simulink model "Mux8Bit4To1"  (R2014a)
settings: Solver=ode45  StartTime=0.0  StopTime=10.0  RelTol=1e-3
libraries: hdlsllib x35
settings Model: Creator=you.r  LastModifiedBy=you.r

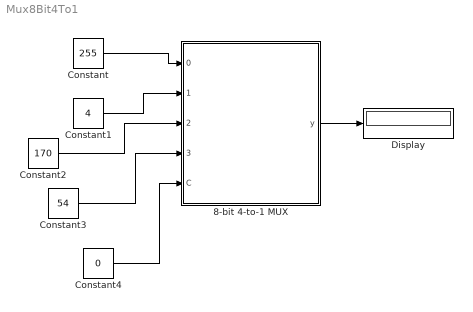
== system Mux8Bit4To1 ==
  8-bit 4-to-1 MUX : Subsystem
  Constant : Constant  Value=255  OutDataTypeStr=uint8  SampleTime=1
  Constant1 : Constant  Value=4  OutDataTypeStr=uint8  SampleTime=1
  Constant2 : Constant  Value=170  OutDataTypeStr=uint8  SampleTime=1
  Constant3 : Constant  Value=54  OutDataTypeStr=uint8  SampleTime=1
  Constant4 : Constant  Value=0  OutDataTypeStr=uint8  SampleTime=1
  Display : Display
  wires:
  Constant/1 -> 8-bit 4-to-1 MUX/1(0)
  Constant1/1 -> 8-bit 4-to-1 MUX/2(1)
  Constant2/1 -> 8-bit 4-to-1 MUX/3(2)
  Constant3/1 -> 8-bit 4-to-1 MUX/4(3)
  Constant4/1 -> 8-bit 4-to-1 MUX/5(C)
  8-bit 4-to-1 MUX/1(y) -> Display/1

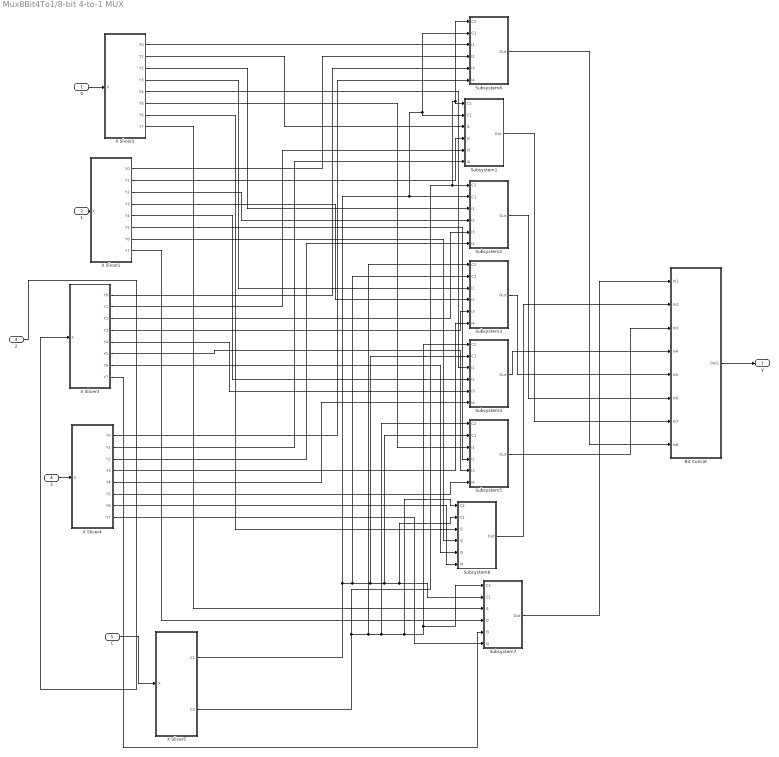
== system Mux8Bit4To1/8-bit 4-to-1 MUX ==
  0 : Inport  OutDataTypeStr=uint8  SampleTime=1
  1 : Inport  Port=2  OutDataTypeStr=uint8  SampleTime=1
  2 : Inport  Port=3  OutDataTypeStr=uint8  SampleTime=1
  3 : Inport  Port=4  OutDataTypeStr=uint8  SampleTime=1
  C : Inport  Port=5  OutDataTypeStr=uint8  SampleTime=1
  Bit Concat : Subsystem
  Subsystem1 : Subsystem
  Subsystem2 : Subsystem
  Subsystem3 : Subsystem
  Subsystem4 : Subsystem
  Subsystem5 : Subsystem
  Subsystem6 : Subsystem
  Subsystem7 : Subsystem
  Subsystem8 : Subsystem
  X Slicer1 : Subsystem
  X Slicer2 : Subsystem
  X Slicer3 : Subsystem
  X Slicer4 : Subsystem
  X Slicer5 : Subsystem
  y : Outport  SampleTime=1
  wires:
  X Slicer1/4(Y3) -> Subsystem3/4(I2)
  1/1 -> X Slicer1/1(X)
  X Slicer3/2(Y1) -> Subsystem1/5(I3)
  X Slicer4/4(Y3) -> Subsystem3/6(I4)
  X Slicer1/1(Y0) -> Subsystem8/4(I2)
  X Slicer1/2(Y1) -> Subsystem1/4(I2)
  X Slicer2/3(Y2) -> Subsystem2/3(I1)
  X Slicer5/2(C2) -> Subsystem2/1(C2), Subsystem1/1(C2), Subsystem8/1(C2), Subsystem3/1(C2), Subsystem5/1(C2), Subsystem6/1(C2), Subsystem7/1(C2), Subsystem4/1(C2)
  X Slicer1/3(Y2) -> Subsystem2/4(I2)
  X Slicer3/7(Y6) -> Subsystem6/5(I3)
  X Slicer2/2(Y1) -> Subsystem1/3(I1)
  X Slicer5/1(C1) -> Subsystem2/2(C1), Subsystem1/2(C1), Subsystem8/2(C1), Subsystem3/2(C1), Subsystem4/2(C1), Subsystem5/2(C1), Subsystem7/2(C1), Subsystem6/2(C1)
  X Slicer4/1(Y0) -> Subsystem8/6(I4)
  0/1 -> X Slicer2/1(X)
  X Slicer3/1(Y0) -> Subsystem8/5(I3)
  X Slicer1/8(Y7) -> Subsystem7/4(I2)
  X Slicer1/5(Y4) -> Subsystem4/4(I2)
  X Slicer3/6(Y5) -> Subsystem5/5(I3)
  X Slicer4/2(Y1) -> Subsystem1/6(I4)
  X Slicer2/6(Y5) -> Subsystem5/3(I1)
  X Slicer4/6(Y5) -> Subsystem5/6(I4)
  X Slicer1/6(Y5) -> Subsystem5/4(I2)
  X Slicer2/1(Y0) -> Subsystem8/3(I1)
  X Slicer4/3(Y2) -> Subsystem2/6(I4)
  X Slicer2/5(Y4) -> Subsystem4/3(I1)
  2/1 -> X Slicer3/1(X)
  3/1 -> X Slicer4/1(X)
  X Slicer1/7(Y6) -> Subsystem6/4(I2)
  Bit Concat/1(Out1) -> y/1
  X Slicer4/7(Y6) -> Subsystem6/6(I4)
  X Slicer3/5(Y4) -> Subsystem4/5(I3)
  X Slicer2/7(Y6) -> Subsystem6/3(I1)
  C/1 -> X Slicer5/1(X)
  X Slicer2/4(Y3) -> Subsystem3/3(I1)
  X Slicer4/5(Y4) -> Subsystem4/6(I4)
  X Slicer3/4(Y3) -> Subsystem3/5(I3)
  X Slicer4/8(Y7) -> Subsystem7/6(I4)
  X Slicer3/8(Y7) -> Subsystem7/5(I3)
  Subsystem2/1(Out) -> Bit Concat/6(In6)
  Subsystem1/1(Out) -> Bit Concat/7(In7)
  Subsystem8/1(Out) -> Bit Concat/8(In8)
  Subsystem3/1(Out) -> Bit Concat/5(In5)
  Subsystem6/1(Out) -> Bit Concat/2(In2)
  Subsystem4/1(Out) -> Bit Concat/4(In4)
  Subsystem5/1(Out) -> Bit Concat/3(In3)
  Subsystem7/1(Out) -> Bit Concat/1(In1)
  X Slicer2/8(Y7) -> Subsystem7/3(I1)
  X Slicer3/3(Y2) -> Subsystem2/5(I3)

== system Mux8Bit4To1/8-bit 4-to-1 MUX/Bit Concat ==
  In1 : Inport
  In2 : Inport  Port=2
  In3 : Inport  Port=3
  In4 : Inport  Port=4
  In5 : Inport  Port=5
  In6 : Inport  Port=6
  In7 : Inport  Port=7
  In8 : Inport  Port=8
  Bit Concat : hdlsllib/HDL Operations/Bit Concat  numInputs=8
  Data Type Conversion : DataTypeConversion  OutDataTypeStr=uint16
  Out1 : Outport
  wires:
  Data Type Conversion/1 -> Out1/1
  Bit Concat/1 -> Data Type Conversion/1
  In7/1 -> Bit Concat/7
  In1/1 -> Bit Concat/1
  In8/1 -> Bit Concat/8
  In6/1 -> Bit Concat/6
  In2/1 -> Bit Concat/2
  In5/1 -> Bit Concat/5
  In3/1 -> Bit Concat/3
  In4/1 -> Bit Concat/4

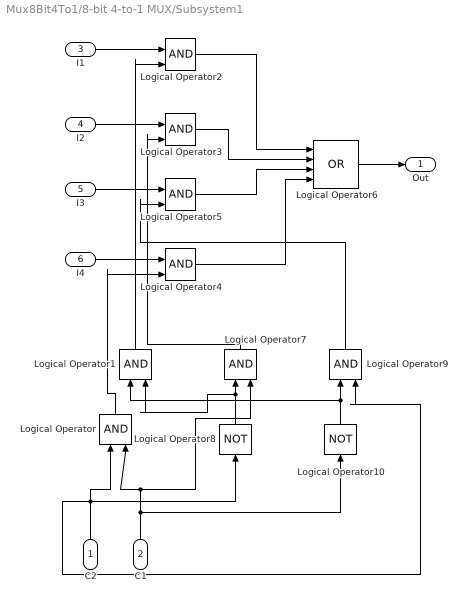
== system Mux8Bit4To1/8-bit 4-to-1 MUX/Subsystem1 ==
  C2 : Inport
  C1 : Inport  Port=2
  I1 : Inport  Port=3
  I2 : Inport  Port=4
  I3 : Inport  Port=5
  I4 : Inport  Port=6
  Logical Operator{,1..5,7,9} (8 alike) : Logic  IconShape=distinctive  AllPortsSameDT=off  OutDataTypeStr=boolean
  Logical Operator10 : Logic  Operator=NOT  IconShape=distinctive  AllPortsSameDT=off  OutDataTypeStr=boolean
  Logical Operator6 : Logic  Operator=OR  Inputs=4  IconShape=distinctive  AllPortsSameDT=off  OutDataTypeStr=boolean
  Logical Operator8 : Logic  Operator=NOT  IconShape=distinctive  AllPortsSameDT=off  OutDataTypeStr=boolean
  Out : Outport
  wires:
  I1/1 -> Logical Operator2/1
  I3/1 -> Logical Operator5/1
  Logical Operator4/1 -> Logical Operator6/4
  Logical Operator3/1 -> Logical Operator6/2
  C1/1 -> Logical Operator10/1, Logical Operator/2, Logical Operator7/2
  C2/1 -> Logical Operator9/2, Logical Operator/1, Logical Operator8/1
  Logical Operator10/1 -> Logical Operator1/1, Logical Operator9/1
  Logical Operator/1 -> Logical Operator4/2
  Logical Operator7/1 -> Logical Operator3/2
  I2/1 -> Logical Operator3/1
  Logical Operator2/1 -> Logical Operator6/1
  Logical Operator9/1 -> Logical Operator5/2
  I4/1 -> Logical Operator4/1
  Logical Operator5/1 -> Logical Operator6/3
  Logical Operator6/1 -> Out/1
  Logical Operator8/1 -> Logical Operator1/2, Logical Operator7/1
  Logical Operator1/1 -> Logical Operator2/2

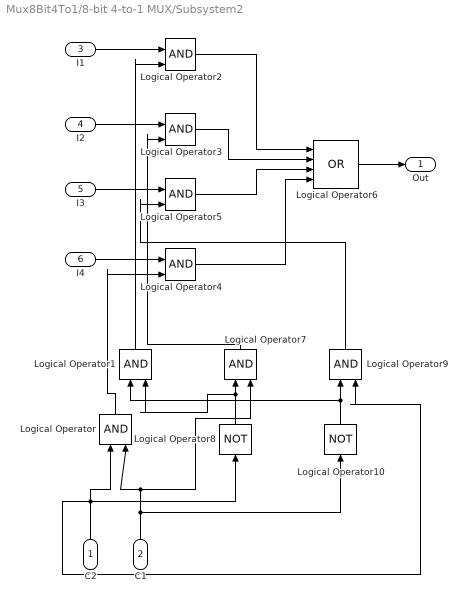
== system Mux8Bit4To1/8-bit 4-to-1 MUX/Subsystem2 ==
  C2 : Inport
  C1 : Inport  Port=2
  I1 : Inport  Port=3
  I2 : Inport  Port=4
  I3 : Inport  Port=5
  I4 : Inport  Port=6
  Logical Operator{,1..5,7,9} (8 alike) : Logic  IconShape=distinctive  AllPortsSameDT=off  OutDataTypeStr=boolean
  Logical Operator10 : Logic  Operator=NOT  IconShape=distinctive  AllPortsSameDT=off  OutDataTypeStr=boolean
  Logical Operator6 : Logic  Operator=OR  Inputs=4  IconShape=distinctive  AllPortsSameDT=off  OutDataTypeStr=boolean
  Logical Operator8 : Logic  Operator=NOT  IconShape=distinctive  AllPortsSameDT=off  OutDataTypeStr=boolean
  Out : Outport
  wires:
  I1/1 -> Logical Operator2/1
  I3/1 -> Logical Operator5/1
  Logical Operator4/1 -> Logical Operator6/4
  Logical Operator3/1 -> Logical Operator6/2
  C1/1 -> Logical Operator10/1, Logical Operator/2, Logical Operator7/2
  C2/1 -> Logical Operator9/2, Logical Operator/1, Logical Operator8/1
  Logical Operator10/1 -> Logical Operator1/1, Logical Operator9/1
  Logical Operator/1 -> Logical Operator4/2
  Logical Operator7/1 -> Logical Operator3/2
  I2/1 -> Logical Operator3/1
  Logical Operator2/1 -> Logical Operator6/1
  Logical Operator9/1 -> Logical Operator5/2
  I4/1 -> Logical Operator4/1
  Logical Operator5/1 -> Logical Operator6/3
  Logical Operator6/1 -> Out/1
  Logical Operator8/1 -> Logical Operator1/2, Logical Operator7/1
  Logical Operator1/1 -> Logical Operator2/2

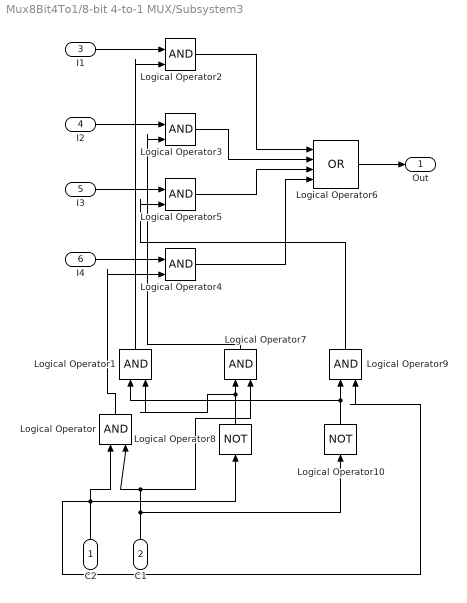
== system Mux8Bit4To1/8-bit 4-to-1 MUX/Subsystem3 ==
  C2 : Inport
  C1 : Inport  Port=2
  I1 : Inport  Port=3
  I2 : Inport  Port=4
  I3 : Inport  Port=5
  I4 : Inport  Port=6
  Logical Operator{,1..5,7,9} (8 alike) : Logic  IconShape=distinctive  AllPortsSameDT=off  OutDataTypeStr=boolean
  Logical Operator10 : Logic  Operator=NOT  IconShape=distinctive  AllPortsSameDT=off  OutDataTypeStr=boolean
  Logical Operator6 : Logic  Operator=OR  Inputs=4  IconShape=distinctive  AllPortsSameDT=off  OutDataTypeStr=boolean
  Logical Operator8 : Logic  Operator=NOT  IconShape=distinctive  AllPortsSameDT=off  OutDataTypeStr=boolean
  Out : Outport
  wires:
  I1/1 -> Logical Operator2/1
  I3/1 -> Logical Operator5/1
  Logical Operator4/1 -> Logical Operator6/4
  Logical Operator3/1 -> Logical Operator6/2
  C1/1 -> Logical Operator10/1, Logical Operator/2, Logical Operator7/2
  C2/1 -> Logical Operator9/2, Logical Operator/1, Logical Operator8/1
  Logical Operator10/1 -> Logical Operator1/1, Logical Operator9/1
  Logical Operator/1 -> Logical Operator4/2
  Logical Operator7/1 -> Logical Operator3/2
  I2/1 -> Logical Operator3/1
  Logical Operator2/1 -> Logical Operator6/1
  Logical Operator9/1 -> Logical Operator5/2
  I4/1 -> Logical Operator4/1
  Logical Operator5/1 -> Logical Operator6/3
  Logical Operator6/1 -> Out/1
  Logical Operator8/1 -> Logical Operator1/2, Logical Operator7/1
  Logical Operator1/1 -> Logical Operator2/2

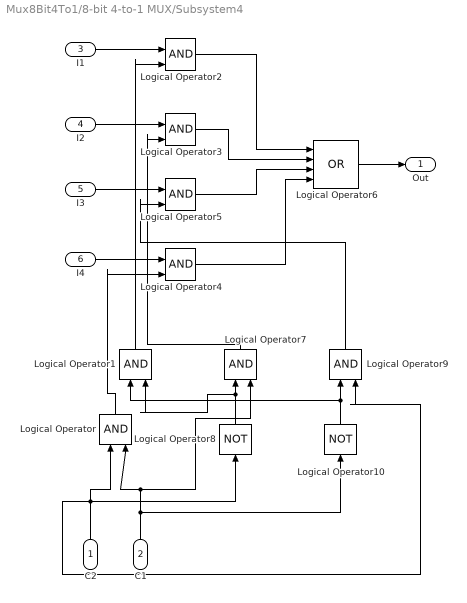
== system Mux8Bit4To1/8-bit 4-to-1 MUX/Subsystem4 ==
  C2 : Inport
  C1 : Inport  Port=2
  I1 : Inport  Port=3
  I2 : Inport  Port=4
  I3 : Inport  Port=5
  I4 : Inport  Port=6
  Logical Operator{,1..5,7,9} (8 alike) : Logic  IconShape=distinctive  AllPortsSameDT=off  OutDataTypeStr=boolean
  Logical Operator10 : Logic  Operator=NOT  IconShape=distinctive  AllPortsSameDT=off  OutDataTypeStr=boolean
  Logical Operator6 : Logic  Operator=OR  Inputs=4  IconShape=distinctive  AllPortsSameDT=off  OutDataTypeStr=boolean
  Logical Operator8 : Logic  Operator=NOT  IconShape=distinctive  AllPortsSameDT=off  OutDataTypeStr=boolean
  Out : Outport
  wires:
  I1/1 -> Logical Operator2/1
  I3/1 -> Logical Operator5/1
  Logical Operator4/1 -> Logical Operator6/4
  Logical Operator3/1 -> Logical Operator6/2
  C1/1 -> Logical Operator10/1, Logical Operator/2, Logical Operator7/2
  C2/1 -> Logical Operator9/2, Logical Operator/1, Logical Operator8/1
  Logical Operator10/1 -> Logical Operator1/1, Logical Operator9/1
  Logical Operator/1 -> Logical Operator4/2
  Logical Operator7/1 -> Logical Operator3/2
  I2/1 -> Logical Operator3/1
  Logical Operator2/1 -> Logical Operator6/1
  Logical Operator9/1 -> Logical Operator5/2
  I4/1 -> Logical Operator4/1
  Logical Operator5/1 -> Logical Operator6/3
  Logical Operator6/1 -> Out/1
  Logical Operator8/1 -> Logical Operator1/2, Logical Operator7/1
  Logical Operator1/1 -> Logical Operator2/2

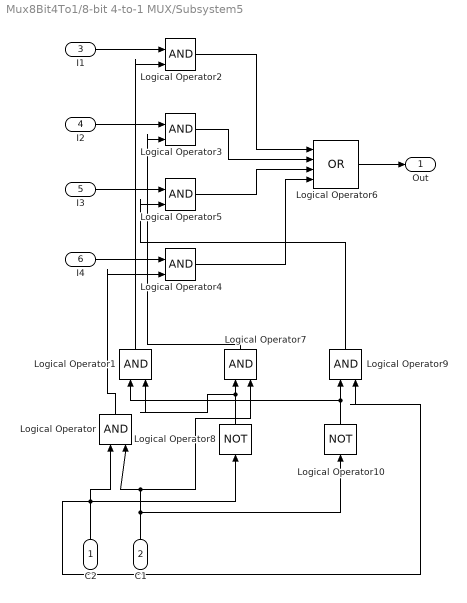
== system Mux8Bit4To1/8-bit 4-to-1 MUX/Subsystem5 ==
  C2 : Inport
  C1 : Inport  Port=2
  I1 : Inport  Port=3
  I2 : Inport  Port=4
  I3 : Inport  Port=5
  I4 : Inport  Port=6
  Logical Operator{,1..5,7,9} (8 alike) : Logic  IconShape=distinctive  AllPortsSameDT=off  OutDataTypeStr=boolean
  Logical Operator10 : Logic  Operator=NOT  IconShape=distinctive  AllPortsSameDT=off  OutDataTypeStr=boolean
  Logical Operator6 : Logic  Operator=OR  Inputs=4  IconShape=distinctive  AllPortsSameDT=off  OutDataTypeStr=boolean
  Logical Operator8 : Logic  Operator=NOT  IconShape=distinctive  AllPortsSameDT=off  OutDataTypeStr=boolean
  Out : Outport
  wires:
  I1/1 -> Logical Operator2/1
  I3/1 -> Logical Operator5/1
  Logical Operator4/1 -> Logical Operator6/4
  Logical Operator3/1 -> Logical Operator6/2
  C1/1 -> Logical Operator10/1, Logical Operator/2, Logical Operator7/2
  C2/1 -> Logical Operator9/2, Logical Operator/1, Logical Operator8/1
  Logical Operator10/1 -> Logical Operator1/1, Logical Operator9/1
  Logical Operator/1 -> Logical Operator4/2
  Logical Operator7/1 -> Logical Operator3/2
  I2/1 -> Logical Operator3/1
  Logical Operator2/1 -> Logical Operator6/1
  Logical Operator9/1 -> Logical Operator5/2
  I4/1 -> Logical Operator4/1
  Logical Operator5/1 -> Logical Operator6/3
  Logical Operator6/1 -> Out/1
  Logical Operator8/1 -> Logical Operator1/2, Logical Operator7/1
  Logical Operator1/1 -> Logical Operator2/2

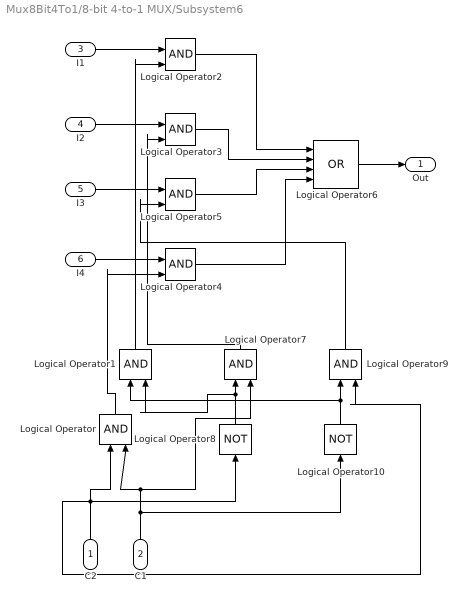
== system Mux8Bit4To1/8-bit 4-to-1 MUX/Subsystem6 ==
  C2 : Inport
  C1 : Inport  Port=2
  I1 : Inport  Port=3
  I2 : Inport  Port=4
  I3 : Inport  Port=5
  I4 : Inport  Port=6
  Logical Operator{,1..5,7,9} (8 alike) : Logic  IconShape=distinctive  AllPortsSameDT=off  OutDataTypeStr=boolean
  Logical Operator10 : Logic  Operator=NOT  IconShape=distinctive  AllPortsSameDT=off  OutDataTypeStr=boolean
  Logical Operator6 : Logic  Operator=OR  Inputs=4  IconShape=distinctive  AllPortsSameDT=off  OutDataTypeStr=boolean
  Logical Operator8 : Logic  Operator=NOT  IconShape=distinctive  AllPortsSameDT=off  OutDataTypeStr=boolean
  Out : Outport
  wires:
  I1/1 -> Logical Operator2/1
  I3/1 -> Logical Operator5/1
  Logical Operator4/1 -> Logical Operator6/4
  Logical Operator3/1 -> Logical Operator6/2
  C1/1 -> Logical Operator10/1, Logical Operator/2, Logical Operator7/2
  C2/1 -> Logical Operator9/2, Logical Operator/1, Logical Operator8/1
  Logical Operator10/1 -> Logical Operator1/1, Logical Operator9/1
  Logical Operator/1 -> Logical Operator4/2
  Logical Operator7/1 -> Logical Operator3/2
  I2/1 -> Logical Operator3/1
  Logical Operator2/1 -> Logical Operator6/1
  Logical Operator9/1 -> Logical Operator5/2
  I4/1 -> Logical Operator4/1
  Logical Operator5/1 -> Logical Operator6/3
  Logical Operator6/1 -> Out/1
  Logical Operator8/1 -> Logical Operator1/2, Logical Operator7/1
  Logical Operator1/1 -> Logical Operator2/2

== system Mux8Bit4To1/8-bit 4-to-1 MUX/Subsystem7 ==
  C2 : Inport
  C1 : Inport  Port=2
  I1 : Inport  Port=3
  I2 : Inport  Port=4
  I3 : Inport  Port=5
  I4 : Inport  Port=6
  Logical Operator{,1..5,7,9} (8 alike) : Logic  IconShape=distinctive  AllPortsSameDT=off  OutDataTypeStr=boolean
  Logical Operator10 : Logic  Operator=NOT  IconShape=distinctive  AllPortsSameDT=off  OutDataTypeStr=boolean
  Logical Operator6 : Logic  Operator=OR  Inputs=4  IconShape=distinctive  AllPortsSameDT=off  OutDataTypeStr=boolean
  Logical Operator8 : Logic  Operator=NOT  IconShape=distinctive  AllPortsSameDT=off  OutDataTypeStr=boolean
  Out : Outport
  wires:
  I1/1 -> Logical Operator2/1
  I3/1 -> Logical Operator5/1
  Logical Operator4/1 -> Logical Operator6/4
  Logical Operator3/1 -> Logical Operator6/2
  C1/1 -> Logical Operator10/1, Logical Operator/2, Logical Operator7/2
  C2/1 -> Logical Operator9/2, Logical Operator/1, Logical Operator8/1
  Logical Operator10/1 -> Logical Operator1/1, Logical Operator9/1
  Logical Operator/1 -> Logical Operator4/2
  Logical Operator7/1 -> Logical Operator3/2
  I2/1 -> Logical Operator3/1
  Logical Operator2/1 -> Logical Operator6/1
  Logical Operator9/1 -> Logical Operator5/2
  I4/1 -> Logical Operator4/1
  Logical Operator5/1 -> Logical Operator6/3
  Logical Operator6/1 -> Out/1
  Logical Operator8/1 -> Logical Operator1/2, Logical Operator7/1
  Logical Operator1/1 -> Logical Operator2/2

== system Mux8Bit4To1/8-bit 4-to-1 MUX/Subsystem8 ==
  C2 : Inport
  C1 : Inport  Port=2
  I1 : Inport  Port=3
  I2 : Inport  Port=4
  I3 : Inport  Port=5
  I4 : Inport  Port=6
  Logical Operator{,1..5,7,9} (8 alike) : Logic  IconShape=distinctive  AllPortsSameDT=off  OutDataTypeStr=boolean
  Logical Operator10 : Logic  Operator=NOT  IconShape=distinctive  AllPortsSameDT=off  OutDataTypeStr=boolean
  Logical Operator6 : Logic  Operator=OR  Inputs=4  IconShape=distinctive  AllPortsSameDT=off  OutDataTypeStr=boolean
  Logical Operator8 : Logic  Operator=NOT  IconShape=distinctive  AllPortsSameDT=off  OutDataTypeStr=boolean
  Out : Outport
  wires:
  I1/1 -> Logical Operator2/1
  I3/1 -> Logical Operator5/1
  Logical Operator4/1 -> Logical Operator6/4
  Logical Operator3/1 -> Logical Operator6/2
  C1/1 -> Logical Operator10/1, Logical Operator/2, Logical Operator7/2
  C2/1 -> Logical Operator9/2, Logical Operator/1, Logical Operator8/1
  Logical Operator10/1 -> Logical Operator1/1, Logical Operator9/1
  Logical Operator/1 -> Logical Operator4/2
  Logical Operator7/1 -> Logical Operator3/2
  I2/1 -> Logical Operator3/1
  Logical Operator2/1 -> Logical Operator6/1
  Logical Operator9/1 -> Logical Operator5/2
  I4/1 -> Logical Operator4/1
  Logical Operator5/1 -> Logical Operator6/3
  Logical Operator6/1 -> Out/1
  Logical Operator8/1 -> Logical Operator1/2, Logical Operator7/1
  Logical Operator1/1 -> Logical Operator2/2

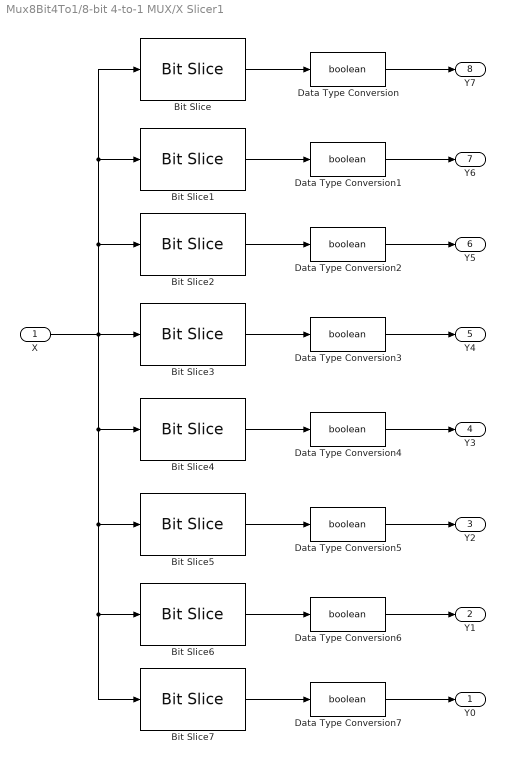
== system Mux8Bit4To1/8-bit 4-to-1 MUX/X Slicer1 ==
  X : Inport  OutDataTypeStr=uint8  SampleTime=1
  Bit Slice : hdlsllib/HDL Operations/Bit Slice  lidx=7  ridx=7
  Bit Slice1 : hdlsllib/HDL Operations/Bit Slice  lidx=6  ridx=6
  Bit Slice2 : hdlsllib/HDL Operations/Bit Slice  lidx=5  ridx=5
  Bit Slice3 : hdlsllib/HDL Operations/Bit Slice  lidx=4  ridx=4
  Bit Slice4 : hdlsllib/HDL Operations/Bit Slice  lidx=3  ridx=3
  Bit Slice5 : hdlsllib/HDL Operations/Bit Slice  lidx=2  ridx=2
  Bit Slice6 : hdlsllib/HDL Operations/Bit Slice  lidx=1  ridx=1
  Bit Slice7 : hdlsllib/HDL Operations/Bit Slice  lidx=0  ridx=0
  Data Type Conversion{,1..7} (8 alike) : DataTypeConversion  OutDataTypeStr=boolean
  Y0 : Outport  OutDataTypeStr=boolean  SampleTime=1
  Y1 : Outport  Port=2  OutDataTypeStr=boolean  SampleTime=1
  Y2 : Outport  Port=3  OutDataTypeStr=boolean  SampleTime=1
  Y3 : Outport  Port=4  OutDataTypeStr=boolean  SampleTime=1
  Y4 : Outport  Port=5  OutDataTypeStr=boolean  SampleTime=1
  Y5 : Outport  Port=6  OutDataTypeStr=boolean  SampleTime=1
  Y6 : Outport  Port=7  OutDataTypeStr=boolean  SampleTime=1
  Y7 : Outport  Port=8  OutDataTypeStr=boolean  SampleTime=1
  wires:
  X/1 -> Bit Slice4/1, Bit Slice5/1, Bit Slice6/1, Bit Slice7/1, Bit Slice3/1, Bit Slice2/1, Bit Slice1/1, Bit Slice/1
  Data Type Conversion/1 -> Y7/1
  Data Type Conversion1/1 -> Y6/1
  Bit Slice2/1 -> Data Type Conversion2/1
  Bit Slice3/1 -> Data Type Conversion3/1
  Bit Slice4/1 -> Data Type Conversion4/1
  Data Type Conversion6/1 -> Y1/1
  Bit Slice/1 -> Data Type Conversion/1
  Bit Slice1/1 -> Data Type Conversion1/1
  Bit Slice6/1 -> Data Type Conversion6/1
  Data Type Conversion7/1 -> Y0/1
  Bit Slice7/1 -> Data Type Conversion7/1
  Bit Slice5/1 -> Data Type Conversion5/1
  Data Type Conversion2/1 -> Y5/1
  Data Type Conversion3/1 -> Y4/1
  Data Type Conversion4/1 -> Y3/1
  Data Type Conversion5/1 -> Y2/1

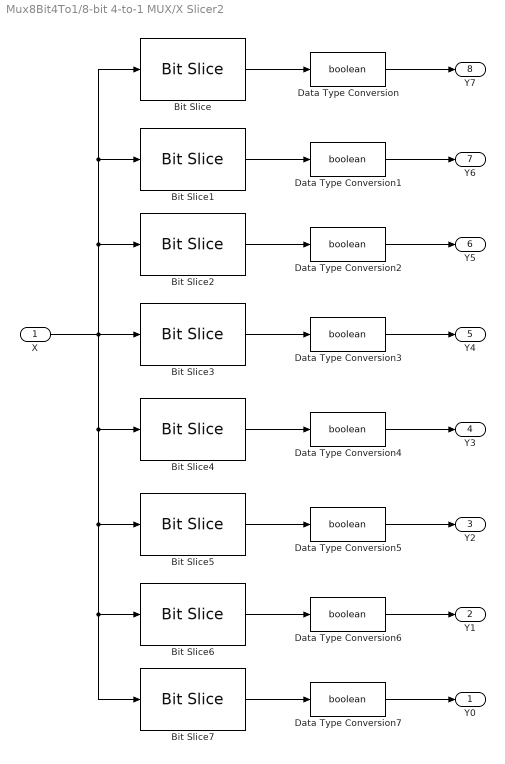
== system Mux8Bit4To1/8-bit 4-to-1 MUX/X Slicer2 ==
  X : Inport  OutDataTypeStr=uint8  SampleTime=1
  Bit Slice : hdlsllib/HDL Operations/Bit Slice  lidx=7  ridx=7
  Bit Slice1 : hdlsllib/HDL Operations/Bit Slice  lidx=6  ridx=6
  Bit Slice2 : hdlsllib/HDL Operations/Bit Slice  lidx=5  ridx=5
  Bit Slice3 : hdlsllib/HDL Operations/Bit Slice  lidx=4  ridx=4
  Bit Slice4 : hdlsllib/HDL Operations/Bit Slice  lidx=3  ridx=3
  Bit Slice5 : hdlsllib/HDL Operations/Bit Slice  lidx=2  ridx=2
  Bit Slice6 : hdlsllib/HDL Operations/Bit Slice  lidx=1  ridx=1
  Bit Slice7 : hdlsllib/HDL Operations/Bit Slice  lidx=0  ridx=0
  Data Type Conversion{,1..7} (8 alike) : DataTypeConversion  OutDataTypeStr=boolean
  Y0 : Outport  OutDataTypeStr=boolean  SampleTime=1
  Y1 : Outport  Port=2  OutDataTypeStr=boolean  SampleTime=1
  Y2 : Outport  Port=3  OutDataTypeStr=boolean  SampleTime=1
  Y3 : Outport  Port=4  OutDataTypeStr=boolean  SampleTime=1
  Y4 : Outport  Port=5  OutDataTypeStr=boolean  SampleTime=1
  Y5 : Outport  Port=6  OutDataTypeStr=boolean  SampleTime=1
  Y6 : Outport  Port=7  OutDataTypeStr=boolean  SampleTime=1
  Y7 : Outport  Port=8  OutDataTypeStr=boolean  SampleTime=1
  wires:
  X/1 -> Bit Slice4/1, Bit Slice5/1, Bit Slice6/1, Bit Slice7/1, Bit Slice3/1, Bit Slice2/1, Bit Slice1/1, Bit Slice/1
  Data Type Conversion/1 -> Y7/1
  Data Type Conversion1/1 -> Y6/1
  Bit Slice2/1 -> Data Type Conversion2/1
  Bit Slice3/1 -> Data Type Conversion3/1
  Bit Slice4/1 -> Data Type Conversion4/1
  Data Type Conversion6/1 -> Y1/1
  Bit Slice/1 -> Data Type Conversion/1
  Bit Slice1/1 -> Data Type Conversion1/1
  Bit Slice6/1 -> Data Type Conversion6/1
  Data Type Conversion7/1 -> Y0/1
  Bit Slice7/1 -> Data Type Conversion7/1
  Bit Slice5/1 -> Data Type Conversion5/1
  Data Type Conversion2/1 -> Y5/1
  Data Type Conversion3/1 -> Y4/1
  Data Type Conversion4/1 -> Y3/1
  Data Type Conversion5/1 -> Y2/1

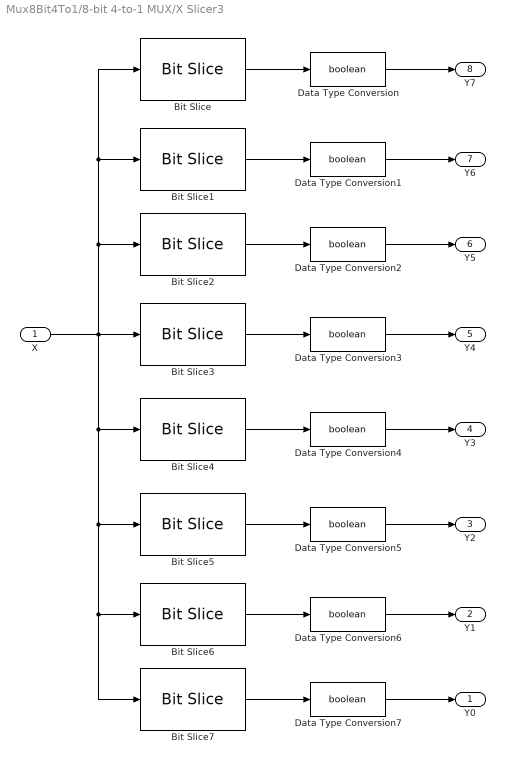
== system Mux8Bit4To1/8-bit 4-to-1 MUX/X Slicer3 ==
  X : Inport  OutDataTypeStr=uint8  SampleTime=1
  Bit Slice : hdlsllib/HDL Operations/Bit Slice  lidx=7  ridx=7
  Bit Slice1 : hdlsllib/HDL Operations/Bit Slice  lidx=6  ridx=6
  Bit Slice2 : hdlsllib/HDL Operations/Bit Slice  lidx=5  ridx=5
  Bit Slice3 : hdlsllib/HDL Operations/Bit Slice  lidx=4  ridx=4
  Bit Slice4 : hdlsllib/HDL Operations/Bit Slice  lidx=3  ridx=3
  Bit Slice5 : hdlsllib/HDL Operations/Bit Slice  lidx=2  ridx=2
  Bit Slice6 : hdlsllib/HDL Operations/Bit Slice  lidx=1  ridx=1
  Bit Slice7 : hdlsllib/HDL Operations/Bit Slice  lidx=0  ridx=0
  Data Type Conversion{,1..7} (8 alike) : DataTypeConversion  OutDataTypeStr=boolean
  Y0 : Outport  OutDataTypeStr=boolean  SampleTime=1
  Y1 : Outport  Port=2  OutDataTypeStr=boolean  SampleTime=1
  Y2 : Outport  Port=3  OutDataTypeStr=boolean  SampleTime=1
  Y3 : Outport  Port=4  OutDataTypeStr=boolean  SampleTime=1
  Y4 : Outport  Port=5  OutDataTypeStr=boolean  SampleTime=1
  Y5 : Outport  Port=6  OutDataTypeStr=boolean  SampleTime=1
  Y6 : Outport  Port=7  OutDataTypeStr=boolean  SampleTime=1
  Y7 : Outport  Port=8  OutDataTypeStr=boolean  SampleTime=1
  wires:
  X/1 -> Bit Slice4/1, Bit Slice5/1, Bit Slice6/1, Bit Slice7/1, Bit Slice3/1, Bit Slice2/1, Bit Slice1/1, Bit Slice/1
  Data Type Conversion/1 -> Y7/1
  Data Type Conversion1/1 -> Y6/1
  Bit Slice2/1 -> Data Type Conversion2/1
  Bit Slice3/1 -> Data Type Conversion3/1
  Bit Slice4/1 -> Data Type Conversion4/1
  Data Type Conversion6/1 -> Y1/1
  Bit Slice/1 -> Data Type Conversion/1
  Bit Slice1/1 -> Data Type Conversion1/1
  Bit Slice6/1 -> Data Type Conversion6/1
  Data Type Conversion7/1 -> Y0/1
  Bit Slice7/1 -> Data Type Conversion7/1
  Bit Slice5/1 -> Data Type Conversion5/1
  Data Type Conversion2/1 -> Y5/1
  Data Type Conversion3/1 -> Y4/1
  Data Type Conversion4/1 -> Y3/1
  Data Type Conversion5/1 -> Y2/1

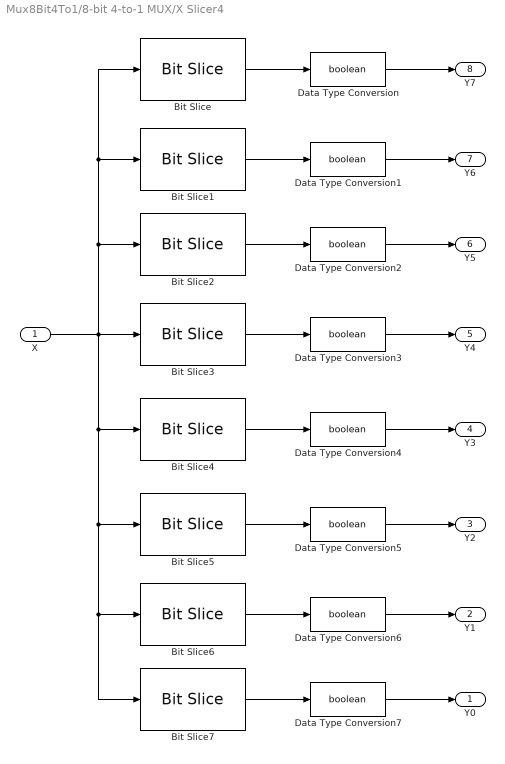
== system Mux8Bit4To1/8-bit 4-to-1 MUX/X Slicer4 ==
  X : Inport  OutDataTypeStr=uint8  SampleTime=1
  Bit Slice : hdlsllib/HDL Operations/Bit Slice  lidx=7  ridx=7
  Bit Slice1 : hdlsllib/HDL Operations/Bit Slice  lidx=6  ridx=6
  Bit Slice2 : hdlsllib/HDL Operations/Bit Slice  lidx=5  ridx=5
  Bit Slice3 : hdlsllib/HDL Operations/Bit Slice  lidx=4  ridx=4
  Bit Slice4 : hdlsllib/HDL Operations/Bit Slice  lidx=3  ridx=3
  Bit Slice5 : hdlsllib/HDL Operations/Bit Slice  lidx=2  ridx=2
  Bit Slice6 : hdlsllib/HDL Operations/Bit Slice  lidx=1  ridx=1
  Bit Slice7 : hdlsllib/HDL Operations/Bit Slice  lidx=0  ridx=0
  Data Type Conversion{,1..7} (8 alike) : DataTypeConversion  OutDataTypeStr=boolean
  Y0 : Outport  OutDataTypeStr=boolean  SampleTime=1
  Y1 : Outport  Port=2  OutDataTypeStr=boolean  SampleTime=1
  Y2 : Outport  Port=3  OutDataTypeStr=boolean  SampleTime=1
  Y3 : Outport  Port=4  OutDataTypeStr=boolean  SampleTime=1
  Y4 : Outport  Port=5  OutDataTypeStr=boolean  SampleTime=1
  Y5 : Outport  Port=6  OutDataTypeStr=boolean  SampleTime=1
  Y6 : Outport  Port=7  OutDataTypeStr=boolean  SampleTime=1
  Y7 : Outport  Port=8  OutDataTypeStr=boolean  SampleTime=1
  wires:
  X/1 -> Bit Slice4/1, Bit Slice5/1, Bit Slice6/1, Bit Slice7/1, Bit Slice3/1, Bit Slice2/1, Bit Slice1/1, Bit Slice/1
  Data Type Conversion/1 -> Y7/1
  Data Type Conversion1/1 -> Y6/1
  Bit Slice2/1 -> Data Type Conversion2/1
  Bit Slice3/1 -> Data Type Conversion3/1
  Bit Slice4/1 -> Data Type Conversion4/1
  Data Type Conversion6/1 -> Y1/1
  Bit Slice/1 -> Data Type Conversion/1
  Bit Slice1/1 -> Data Type Conversion1/1
  Bit Slice6/1 -> Data Type Conversion6/1
  Data Type Conversion7/1 -> Y0/1
  Bit Slice7/1 -> Data Type Conversion7/1
  Bit Slice5/1 -> Data Type Conversion5/1
  Data Type Conversion2/1 -> Y5/1
  Data Type Conversion3/1 -> Y4/1
  Data Type Conversion4/1 -> Y3/1
  Data Type Conversion5/1 -> Y2/1

== system Mux8Bit4To1/8-bit 4-to-1 MUX/X Slicer5 ==
  X : Inport  OutDataTypeStr=uint8  SampleTime=1
  Bit Slice6 : hdlsllib/HDL Operations/Bit Slice  lidx=1  ridx=1
  Bit Slice7 : hdlsllib/HDL Operations/Bit Slice  lidx=0  ridx=0
  Data Type Conversion6 : DataTypeConversion  OutDataTypeStr=boolean
  Data Type Conversion7 : DataTypeConversion  OutDataTypeStr=boolean
  C1 : Outport  OutDataTypeStr=boolean  SampleTime=1
  C2 : Outport  Port=2  OutDataTypeStr=boolean  SampleTime=1
  wires:
  X/1 -> Bit Slice6/1, Bit Slice7/1
  Data Type Conversion6/1 -> C2/1
  Bit Slice6/1 -> Data Type Conversion6/1
  Data Type Conversion7/1 -> C1/1
  Bit Slice7/1 -> Data Type Conversion7/1
